simulink model "quad_input"  (R2017a)
settings: Solver=VariableStepAuto  StartTime=0.0  StopTime=10.0  RelTol=1e-3
libraries: simulink x2
settings Model: Creator=sidag  LastModifiedBy=sidag

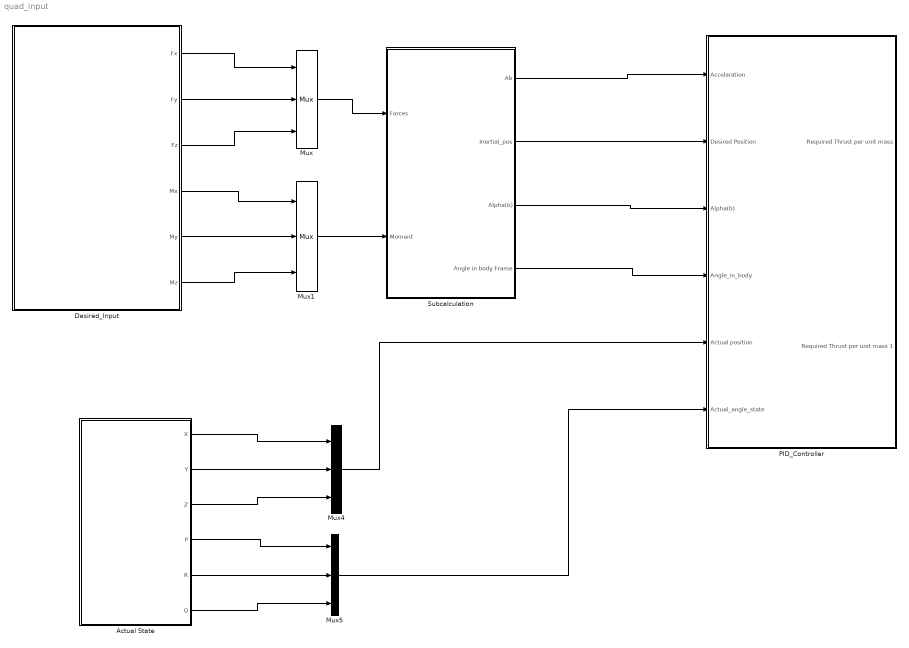
== system quad_input ==
  Actual State : Subsystem
  Desired_Input : Subsystem
  Mux{,1,4..5} (4 alike) : Mux  Inputs=3
  PID_Controller : Subsystem
  Subcalculation : Subsystem
  wires:
  Mux/1 -> Subcalculation/1("Forces ")
  Mux1/1 -> Subcalculation/2(Moment)
  Desired_Input/1(Fx) -> Mux/1
  Desired_Input/2(Fy) -> Mux/2
  Desired_Input/3(Fz) -> Mux/3
  Desired_Input/4(Mx) -> Mux1/1
  Desired_Input/5(My) -> Mux1/2
  Desired_Input/6("Mz ") -> Mux1/3
  Actual State/1(X) -> Mux4/1
  Actual State/2(Y) -> Mux4/2
  Actual State/3(Z) -> Mux4/3
  Actual State/6(Q) -> Mux5/3
  Actual State/5(R) -> Mux5/2
  Actual State/4(P) -> Mux5/1
  Mux4/1 -> PID_Controller/5(Actual position)
  Subcalculation/1("Ab ") -> PID_Controller/1(Accelaration)
  Subcalculation/2(Inertial_pos) -> PID_Controller/2("Desired Position ")
  Mux5/1 -> PID_Controller/6(Actual_angle_state)
  Subcalculation/4(Angle in body Frame) -> PID_Controller/4(Angle_in_body)
  Subcalculation/3("Alpha(b) ") -> PID_Controller/3(Alpha(b))

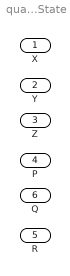
== system quad_input/Actual State ==
  X : Outport
  Y : Outport  Port=2
  Z : Outport  Port=3
  P : Outport  Port=4
  R : Outport  Port=5
  Q : Outport  Port=6

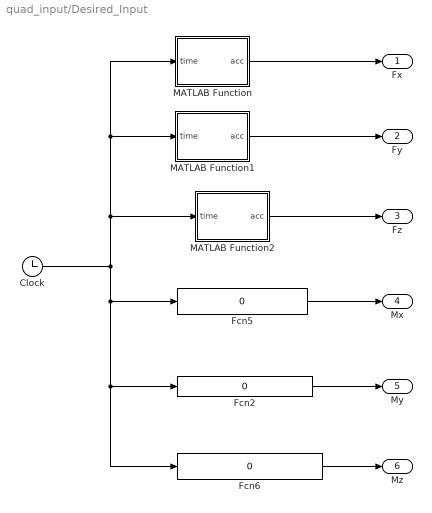
== system quad_input/Desired_Input ==
  Clock : Clock
  Fcn2 : Fcn  Expr=0
  Fcn5 : Fcn  Expr=0
  Fcn6 : Fcn  Expr=0
  MATLAB Function : MATLAB Function  TreatAsAtomicUnit=on
  MATLAB Function1 : MATLAB Function  TreatAsAtomicUnit=on
  MATLAB Function2 : MATLAB Function  TreatAsAtomicUnit=on
  Fx : Outport
  Fy : Outport  Port=2
  Fz : Outport  Port=3
  Mx : Outport  Port=4
  My : Outport  Port=5
  "Mz " : Outport  Port=6
  wires:
  Clock/1 -> Fcn6/1, Fcn2/1, Fcn5/1, MATLAB Function2/1(time), MATLAB Function/1(time), MATLAB Function1/1(time)
  Fcn2/1 -> My/1
  Fcn6/1 -> "Mz "/1
  MATLAB Function2/1(acc) -> Fz/1
  Fcn5/1 -> Mx/1
  MATLAB Function/1(acc) -> Fx/1
  MATLAB Function1/1(acc) -> Fy/1

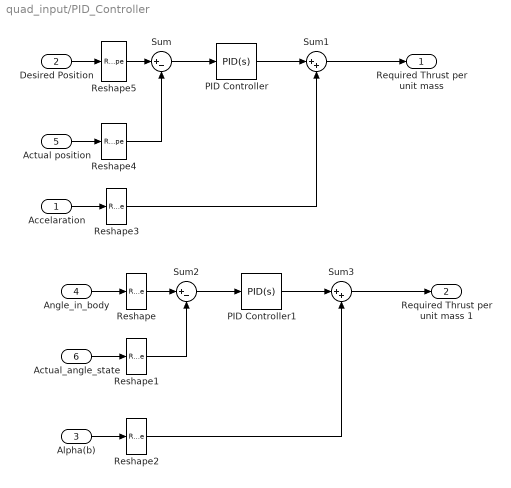
== system quad_input/PID_Controller ==
  Accelaration : Inport
  "Desired Position " : Inport  Port=2
  Alpha(b) : Inport  Port=3
  Angle_in_body : Inport  Port=4
  Actual position : Inport  Port=5
  Actual_angle_state : Inport  Port=6
  PID Controller : simulink/Continuous/PID Controller  Controller=PID  TimeDomain=Continuous-time  SampleTime=-1  IntegratorMethod=Forward Euler  FilterMethod=Forward Euler  Form=Parallel  UseFilter=on  ControllerParametersSource=internal  P=1  I=1  D=0  N=100  InitialConditionSource=internal  InitialConditionForIntegrator=0  InitialConditionForFilter=0  ExternalReset=none  LimitOutput=off  UpperSaturationLimit=inf  LowerSaturationLimit=-inf  LinearizeAsGain=on  AntiWindupMode=none  Kb=1  TrackingMode=off  Kt=1  PParamMin=[]  PParamMax=[]  IParamMin=[]  IParamMax=[]  DParamMin=[]  DParamMax=[]  NParamMin=[]  NParamMax=[]  KbParamMin=[]  KbParamMax=[]  KtParamMin=[]  KtParamMax=[]  POutMin=[]  POutMax=[]  IOutMin=[]  IOutMax=[]  DOutMin=[]  DOutMax=[]  NOutMin=[]  NOutMax=[]  KbOutMin=[]  KbOutMax=[]  KtOutMin=[]  KtOutMax=[]  IntegratorOutMin=[]  IntegratorOutMax=[]  FilterOutMin=[]  FilterOutMax=[]  SumOutMin=[]  SumOutMax=[]  SumI1OutMin=[]  SumI1OutMax=[]  SumI2OutMin=[]  SumI2OutMax=[]  SumI3OutMin=[]  SumI3OutMax=[]  SumDOutMin=[]  SumDOutMax=[]  SaturationOutMin=[]  SaturationOutMax=[]  IntegratorContinuousStateAttributes=''  IntegratorStateMustResolveToSignalObject=off  IntegratorRTWStateStorageClass=Auto  FilterContinuousStateAttributes=''  FilterStateMustResolveToSignalObject=off  FilterRTWStateStorageClass=Auto  DifferentiatorICPrevScaledInput=0  DifferentiatorOutMin=[]  DifferentiatorOutMax=[]  InitialConditionSetting=State (most efficient)
  PID Controller1 : simulink/Continuous/PID Controller  Controller=PID  TimeDomain=Continuous-time  SampleTime=-1  IntegratorMethod=Forward Euler  FilterMethod=Forward Euler  Form=Parallel  UseFilter=on  ControllerParametersSource=internal  P=1  I=1  D=0  N=100  InitialConditionSource=internal  InitialConditionForIntegrator=0  InitialConditionForFilter=0  ExternalReset=none  LimitOutput=off  UpperSaturationLimit=inf  LowerSaturationLimit=-inf  LinearizeAsGain=on  AntiWindupMode=none  Kb=1  TrackingMode=off  Kt=1  PParamMin=[]  PParamMax=[]  IParamMin=[]  IParamMax=[]  DParamMin=[]  DParamMax=[]  NParamMin=[]  NParamMax=[]  KbParamMin=[]  KbParamMax=[]  KtParamMin=[]  KtParamMax=[]  POutMin=[]  POutMax=[]  IOutMin=[]  IOutMax=[]  DOutMin=[]  DOutMax=[]  NOutMin=[]  NOutMax=[]  KbOutMin=[]  KbOutMax=[]  KtOutMin=[]  KtOutMax=[]  IntegratorOutMin=[]  IntegratorOutMax=[]  FilterOutMin=[]  FilterOutMax=[]  SumOutMin=[]  SumOutMax=[]  SumI1OutMin=[]  SumI1OutMax=[]  SumI2OutMin=[]  SumI2OutMax=[]  SumI3OutMin=[]  SumI3OutMax=[]  SumDOutMin=[]  SumDOutMax=[]  SaturationOutMin=[]  SaturationOutMax=[]  IntegratorContinuousStateAttributes=''  IntegratorStateMustResolveToSignalObject=off  IntegratorRTWStateStorageClass=Auto  FilterContinuousStateAttributes=''  FilterStateMustResolveToSignalObject=off  FilterRTWStateStorageClass=Auto  DifferentiatorICPrevScaledInput=0  DifferentiatorOutMin=[]  DifferentiatorOutMax=[]  InitialConditionSetting=State (most efficient)
  Reshape{,1..5} (6 alike) : Reshape  OutputDimensionality=Column vector (2-D)
  Sum : Sum  Inputs=|+-
  Sum1 : Sum  Inputs=|++
  Sum2 : Sum  Inputs=|+-
  Sum3 : Sum  Inputs=|++
  "Required Thrust per unit mass " : Outport
  Required Thrust per unit mass 1 : Outport  Port=2
  wires:
  "Desired Position "/1 -> Reshape5/1
  Actual position/1 -> Reshape4/1
  Sum/1 -> PID Controller/1
  PID Controller/1 -> Sum1/1
  Accelaration/1 -> Reshape3/1
  Sum1/1 -> "Required Thrust per unit mass "/1
  Sum3/1 -> Required Thrust per unit mass 1/1
  Actual_angle_state/1 -> Reshape1/1
  PID Controller1/1 -> Sum3/1
  Sum2/1 -> PID Controller1/1
  Angle_in_body/1 -> Reshape/1
  Alpha(b)/1 -> Reshape2/1
  Reshape/1 -> Sum2/1
  Reshape1/1 -> Sum2/2
  Reshape2/1 -> Sum3/2
  Reshape3/1 -> Sum1/2
  Reshape4/1 -> Sum/2
  Reshape5/1 -> Sum/1

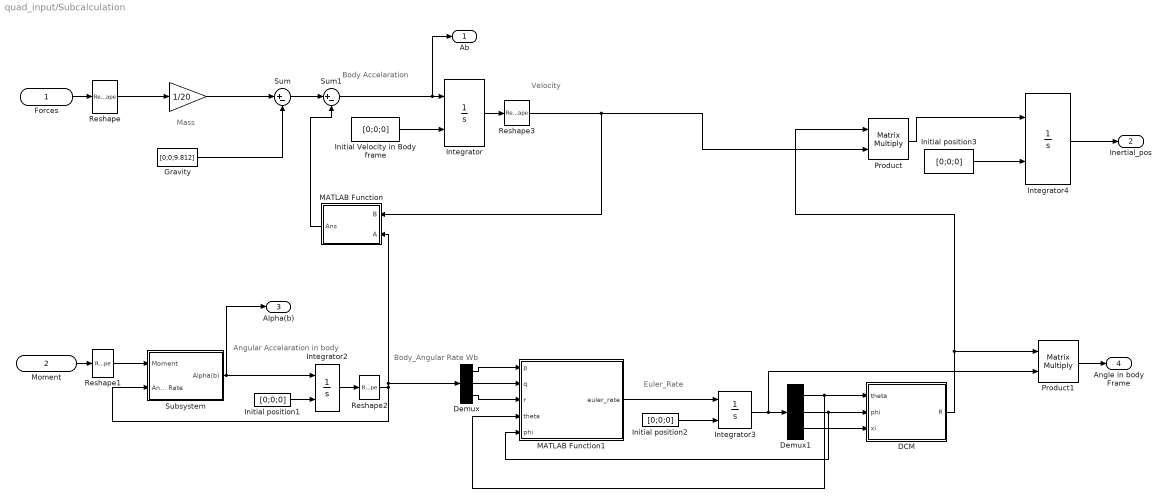
== system quad_input/Subcalculation ==
  note: Angular Accelaration
      | in body
  note: Body_Angular
      | Rate Wb
  note: Euler_Rate
  note: Mass
  note: Velocity
  note: Body Accelaration
  "Forces " : Inport
  Moment : Inport  Port=2
  " " : Gain  Gain=1/20
  DCM : MATLAB Function  TreatAsAtomicUnit=on
  Demux : Demux  Outputs=3
  Demux1 : Demux  Outputs=3
  "Gravity " : Constant  Value=[0;0;9.812]  VectorParams1D=off
  "Initial Velocity in Body frame " : Constant  Value=[0;0;0]
  Initial position1 : Constant  Value=[0;0;0]
  Initial position2 : Constant  Value=[0;0;0]
  Initial position3 : Constant  Value=[0;0;0]
  Integrator{,2..4} (4 alike) : Integrator  InitialConditionSource=external
  MATLAB Function : MATLAB Function  TreatAsAtomicUnit=on
  MATLAB Function1 : MATLAB Function  TreatAsAtomicUnit=on
  Product : Product  Multiplication=Matrix(*)
  Product1 : Product  Multiplication=Matrix(*)
  Reshape{,1..3} (4 alike) : Reshape  OutputDimensionality=Column vector (2-D)
  Subsystem : Subsystem
  Sum : Sum  Inputs=|+-
  Sum1 : Sum  Inputs=|+-
  "Ab " : Outport
  Inertial_pos : Outport  Port=2
  "Alpha(b) " : Outport  Port=3
  Angle in body Frame : Outport  Port=4
  wires:
  "Forces "/1 -> Reshape/1
  " "/1 -> Sum/1
  "Gravity "/1 -> Sum/2
  Sum/1 -> Sum1/1
  MATLAB Function/1(Ans) -> Sum1/2
  Sum1/1 -> "Ab "/1, Integrator/1
  Integrator/1 -> Reshape3/1
  "Initial Velocity in Body frame "/1 -> Integrator/2
  Integrator2/1 -> Reshape2/1
  Moment/1 -> Reshape1/1
  Initial position1/1 -> Integrator2/2
  Subsystem/1(Alpha(b)) -> "Alpha(b) "/1, Integrator2/1
  Demux/1 -> MATLAB Function1/1(p)
  Demux/2 -> MATLAB Function1/2(q)
  Demux/3 -> MATLAB Function1/3(r)
  Initial position2/1 -> Integrator3/2
  MATLAB Function1/1(euler_rate) -> Integrator3/1
  Integrator3/1 -> Product1/2, Demux1/1
  Initial position3/1 -> Integrator4/2
  Product/1 -> Integrator4/1
  Demux1/2 -> MATLAB Function1/5(phi), DCM/2(phi)
  Demux1/3 -> DCM/3(xi)
  Demux1/1 -> MATLAB Function1/4(theta), DCM/1(theta)
  Integrator4/1 -> Inertial_pos/1
  DCM/1(R) -> Product1/1, Product/1
  Reshape/1 -> " "/1
  Reshape1/1 -> Subsystem/1("Moment ")
  Reshape2/1 -> MATLAB Function/2(A), Demux/1, Subsystem/2("Angular Rate ")
  Reshape3/1 -> Product/2, MATLAB Function/1(B)
  Product1/1 -> Angle in body Frame/1

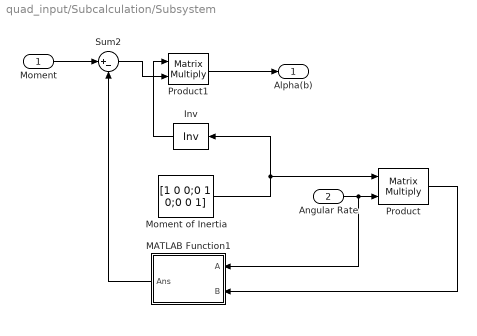
== system quad_input/Subcalculation/Subsystem ==
  "Moment " : Inport
  "Angular Rate " : Inport  Port=2
  Inv : Product  Inputs=/  Multiplication=Matrix(*)
  MATLAB Function1 : MATLAB Function  TreatAsAtomicUnit=on
  "Moment of Inertia " : Constant  Value=[1 0 0;0 1 0;0 0 1]
  Product : Product  Multiplication=Matrix(*)
  Product1 : Product  Multiplication=Matrix(*)
  Sum2 : Sum  Inputs=|+-
  Alpha(b) : Outport
  wires:
  Product/1 -> MATLAB Function1/2(B)
  Sum2/1 -> Product1/2
  Inv/1 -> Product1/1
  "Moment of Inertia "/1 -> Product/1, Inv/1
  "Moment "/1 -> Sum2/1
  MATLAB Function1/1(Ans) -> Sum2/2
  Product1/1 -> Alpha(b)/1
  "Angular Rate "/1 -> Product/2, MATLAB Function1/1(A)

== matlab function quad_input/Subcalculation/MATLAB Function ==
  data: B input; A input; Ans output
function Ans=cross(B,A)
Ahat=[0 -A(3) A(2);A(3) 0 -A(1);-A(2) A(1) 0];
Ans=Ahat*B;
end

== matlab function quad_input/Subcalculation/MATLAB Function1 ==
  data: p input; q input; r input; theta input; euler_rate output; phi input
function euler_rate = euler_rates(p,q,r,theta,phi)
%Under the following condition 
%Euler_rate=[xidot;thetadot;phidot] xidot around x thetadot around y phidot
%around z 
%Rotation is around X-Y-Z axis
%omegahatinertial=Rdot*R';
% Ris Rsb
% A comes from A*euler_rates=omegabody
%omegabody=[p;q;r]
A=[-cos(phi)*cos(theta),sin(phi),0;-cos(theta)*sin(phi),-cos(phi),0;sin(theta),0,-1];
euler_rate=(A)\[p;q;r];
end

== matlab function quad_input/Subcalculation/DCM ==
  data: theta input; phi input; xi input; R output
function R= Rotation(theta,phi,xi)

Rx=[1,0,0;0,cos(xi),-sin(xi);0,sin(xi),cos(xi)]';
Ry=[cos(theta),0,sin(theta);0,1,0;-sin(theta),0,cos(theta)]';
Rz=[cos(phi),-sin(phi),0;sin(phi),cos(phi),0;0,0,1]';
R=(Rx*Ry*Rz);

== matlab function quad_input/Subcalculation/Subsystem/MATLAB Function1 ==
  data: A input; Ans output; B input
function Ans=cross(A,B)
Ahat=[0 -A(3) A(2);A(3) 0 -A(1);-A(2) A(1) 0];
Ans=Ahat*B;
end

== matlab function quad_input/Desired_Input/MATLAB Function ==
  data: time input; acc output
function acc= fcn(time)
acc=0;
if time<=5 
    acc=0;
end

if 5<time&&time<=15
    acc=200;
end
if 15<time&&time<=25
    acc=-200;
end
if 25<time&&time<=30
    acc=0;
end
if 30<time&&time<=40
    acc=200;
end
if 40<time&&time<=50
    acc=-200;
end
if time>50
    acc=0;
end
end

== matlab function quad_input/Desired_Input/MATLAB Function1 ==
  data: time input; acc output
function acc = fcn(time)
acc=0;
if time<=25 
    acc=0;
end

if 25<time&&time<=27.5
    acc=400;
end
if 27.5<time&&time<=30
    acc=-400;
end
if 30<time&&time<=50
    acc=0;
end
if time>50
    acc=0;
end

== matlab function quad_input/Desired_Input/MATLAB Function2 ==
  data: time input; acc output
function acc = fcn(time)
acc=0;
if time<=2.5 
    acc=236.2;
end

if 2.5<time&&time<=5
    acc=-236.2;
end
if 5<time
    acc=196.2;
end

end
